simulink model "gpt_gui"  (R2021b)
settings: Solver=FixedStepAuto  StartTime=0.0  StopTime=20.0  RelTol=1e-3  EnableMultiTasking=on
settings Model: Creator=Thomas  LastModifiedBy=Thomas
settings SolverCC: PositivePriorityOrder=on
settings OptimizationCC: EnhancedBackFolding=on  PassReuseOutputArgsAs=Individual arguments  ZeroExternalMemoryAtStartup=off  ZeroInternalMemoryAtStartup=off  MaxStackSize=64  OptimizeBlockOrder=speed  DifferentSizesBufferReuse=on  OptimizationCustomize=off  EfficientTunableParamExpr=on
settings DebuggingCC: ParameterTunabilityLossMsg=error
settings HardwareCC: ProdBitPerPointer=32  ProdBitPerSizeT=32  ProdBitPerPtrDiffT=32  ProdLargestAtomicInteger=Long  ProdLargestAtomicFloat=Double  ProdWordSize=32  ProdLongLongMode=on  ProdHWDeviceType=ARM Compatible->ARM Cortex  UseEmbeddedCoderFeatures=off  UseSimulinkCoderFeatures=off
settings RTWCC: Description=Embedded Coder  SystemTargetFile=ert.tlc  HardwareBoard=Raspberry Pi  TLCOptions="-aInlineSetEventsForThisBaseRateFcn=TLC_FALSE -aSuppressMultiTaskScheduler=TLC_FALSE  -aRateBasedStepFcn=0"  TemplateMakefile=ert_default_tmf  Toolchain=GNU GCC Embedded Linux  BuildConfiguration=Faster Runs
settings CodeAppCC: ForceParamTrailComments=on  IgnoreCustomStorageClasses=off  OperatorAnnotations=on  SimulinkDataObjDesc=on  SFDataObjDesc=on  InsertBlockDesc=on
settings ERTTargetCC: SupportNonInlinedSFcns=on  SupportVariableSizeSignals=on  ExtModeTransport=2  ExtModeStaticAlloc=on  ExtModeMexFile=ext_xcp  ExtModeIntrfLevel=Level2 - Open

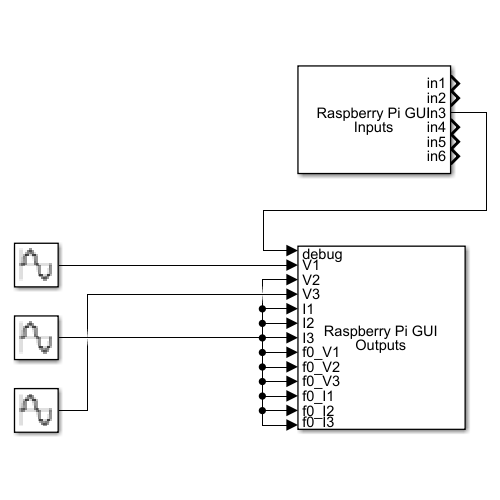
[thumbnail: Simulink's stored preview of the top-level diagram]
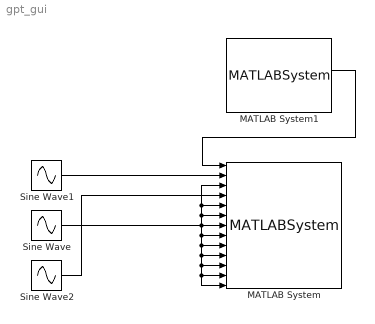
== system gpt_gui ==
  MATLAB System : MATLABSystem  System=GuiOutputs
      mask Type: GuiOutputs
      mask Display:
      | disp('Raspberry Pi GUI\nOutputs');
      | port_label('input',1,'debug');
      | port_label('input',2,'V1');
      | port_label('input',3,'V2');
      | port_label('input',4,'V3');
      | port_label('input',5,'I1');
      | port_label('input',6,'I2');
      | port_label('input',7,'I3');
      | port_label('input',8,'f0_V1');
      | port_label('input',9,'f0_V2');
      | port_label('input',10,'f0_V3');
      | port_label('input',11,'f0_I1');
      | port_label('input',12,'f0_I2');
      | port_label('input',13,'f0_I3');
  MATLAB System1 : MATLABSystem  System=GuiInputs  SampleTime=0.1
      mask Type: GuiInputs
      mask Display:
      | disp('Raspberry Pi GUI\nInputs');
      | port_label('output',1,'in1');
      | port_label('output',2,'in2');
      | port_label('output',3,'in3');
      | port_label('output',4,'in4');
      | port_label('output',5,'in5');
      | port_label('output',6,'in6');
  Sine Wave : Sin  Frequency=2*pi*50  SampleTime=0.001
  Sine Wave1 : Sin  Frequency=2*pi*120  SampleTime=0.001
  Sine Wave2 : Sin  Frequency=2*pi*50  Phase=(60/180)*pi  SampleTime=0.001
  wires:
  Sine Wave/1 -> MATLAB System/7, MATLAB System/8, MATLAB System/9, MATLAB System/10, MATLAB System/11, MATLAB System/12, MATLAB System/13, MATLAB System/6, MATLAB System/5, MATLAB System/3
  MATLAB System1/3 -> MATLAB System/1
  Sine Wave1/1 -> MATLAB System/2
  Sine Wave2/1 -> MATLAB System/4
